simulink model "parallel_force_control_position"  (R2023a)
settings: Solver=VariableStepAuto  StartTime=0.0  StopTime=10.0  RelTol=1e-3
undefined symbols (not defined in the file): dqi, fd, K, KD, KF, KI, KP, Md, qi, robot, xd, xr
settings Model: Creator=franc  LastModifiedBy=franc

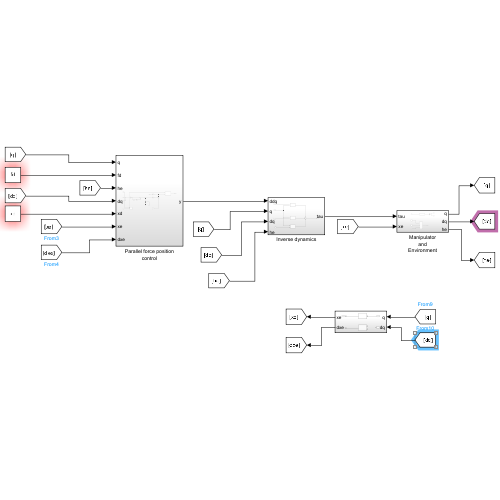
[thumbnail: Simulink's stored preview of the top-level diagram]
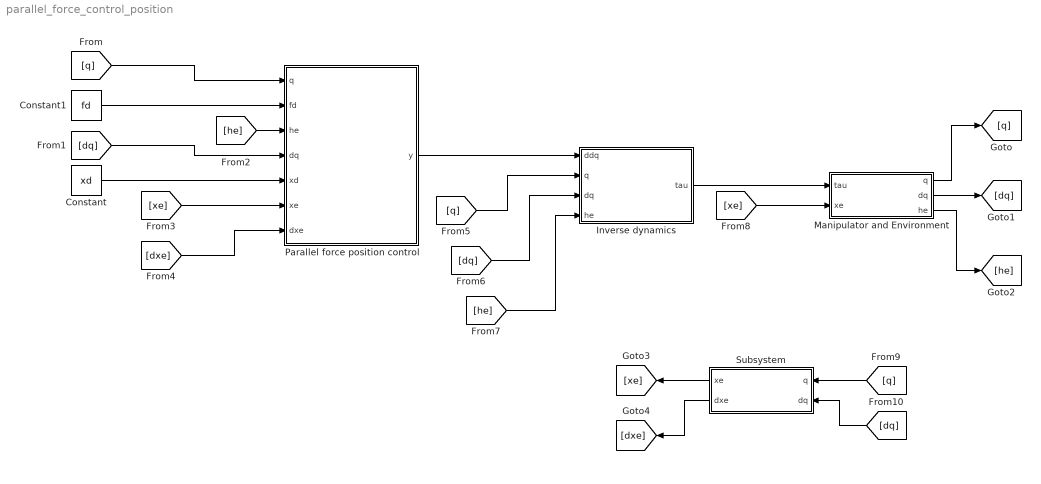
== system parallel_force_control_position ==
  Constant : Constant  Value=xd
  Constant1 : Constant  Value=fd
  Inverse dynamics : Subsystem
  Manipulator and Environment : Subsystem
  Parallel force position control : Subsystem
  Subsystem : Subsystem
  wires:
  Constant/1 -> Parallel force position control/5(xd)
  Constant1/1 -> Parallel force position control/2(fd)
  [q] -> Parallel force position control/1(q)
  [dq] -> Parallel force position control/4(dq)
  [he] -> Parallel force position control/3(he)
  [xe] -> Parallel force position control/6(xe)
  [dxe] -> Parallel force position control/7(dxe)
  Parallel force position control/1(y) -> Inverse dynamics/1(ddq)
  [q] -> Inverse dynamics/2(q)
  [dq] -> Inverse dynamics/3(dq)
  [he] -> Inverse dynamics/4(he)
  Inverse dynamics/1(tau) -> Manipulator and Environment/1(tau)
  [xe] -> Manipulator and Environment/2(xe)
  Manipulator and Environment/1(q) -> [q]
  Manipulator and Environment/2(dq) -> [dq]
  Manipulator and Environment/3(he) -> [he]
  Subsystem/1(xe) -> [xe]
  Subsystem/2(dxe) -> [dxe]
  [dq] -> Subsystem/2(dq)
  [q] -> Subsystem/1(q)

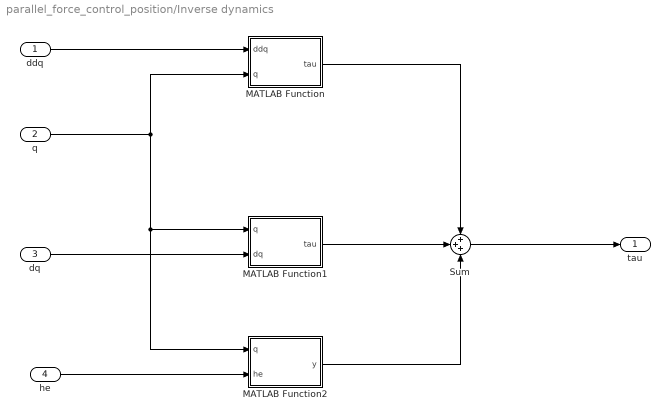
== system parallel_force_control_position/Inverse dynamics ==
  ddq : Inport
  q : Inport  Port=2
  dq : Inport  Port=3
  he : Inport  Port=4
  MATLAB Function : MATLAB Function  TreatAsAtomicUnit=on
  MATLAB Function1 : MATLAB Function  TreatAsAtomicUnit=on
  MATLAB Function2 : MATLAB Function  TreatAsAtomicUnit=on
  Sum : Sum  Inputs=+++
  tau : Outport
  wires:
  ddq/1 -> MATLAB Function/1(ddq)
  q/1 -> MATLAB Function1/1(q), MATLAB Function2/1(q), MATLAB Function/2(q)
  dq/1 -> MATLAB Function1/2(dq)
  he/1 -> MATLAB Function2/2(he)
  MATLAB Function1/1(tau) -> Sum/2
  MATLAB Function/1(tau) -> Sum/1
  MATLAB Function2/1(y) -> Sum/3
  Sum/1 -> tau/1

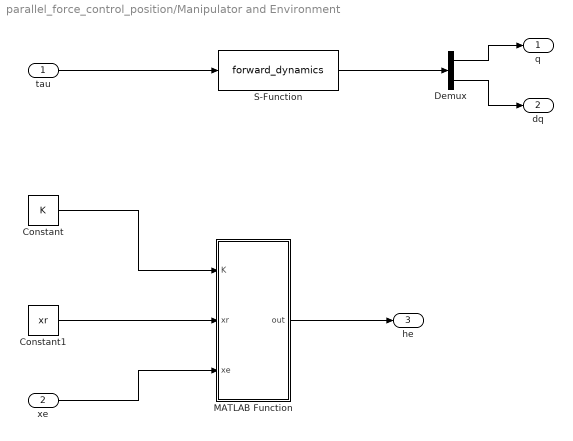
== system parallel_force_control_position/Manipulator and Environment ==
  tau : Inport
  xe : Inport  Port=2
  Constant : Constant  Value=K
  Constant1 : Constant  Value=xr
  Demux : Demux  Outputs=2
  MATLAB Function : MATLAB Function  TreatAsAtomicUnit=on
  S-Function : S-Function  FunctionName=forward_dynamics  Parameters=robot,qi,dqi  SFunctionDeploymentMode=off  EnableBusSupport=off
  q : Outport
  dq : Outport  Port=2
  he : Outport  Port=3
  wires:
  tau/1 -> S-Function/1
  Constant1/1 -> MATLAB Function/2(xr)
  Constant/1 -> MATLAB Function/1(K)
  xe/1 -> MATLAB Function/3(xe)
  MATLAB Function/1(out) -> he/1
  S-Function/1 -> Demux/1
  Demux/1 -> q/1
  Demux/2 -> dq/1

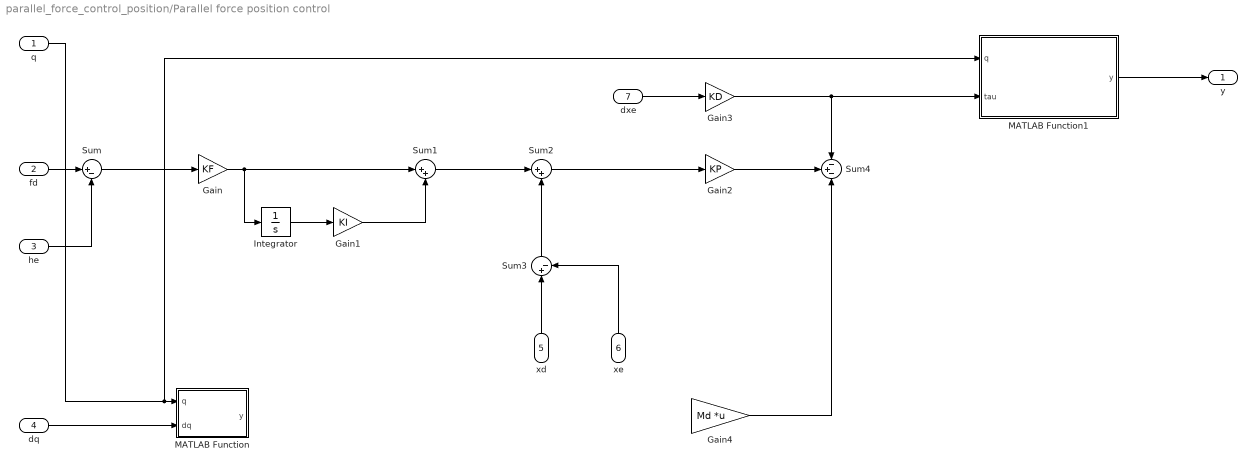
== system parallel_force_control_position/Parallel force position control ==
  q : Inport
  fd : Inport  Port=2
  he : Inport  Port=3
  dq : Inport  Port=4
  xd : Inport  Port=5
  xe : Inport  Port=6
  dxe : Inport  Port=7
  Gain : Gain  Gain=KF
  Gain1 : Gain  Gain=KI
  Gain2 : Gain  Gain=KP
  Gain3 : Gain  Gain=KD
  Gain4 : Gain  Gain=Md  Multiplication=Matrix(K*u)
  Integrator : Integrator
  MATLAB Function : MATLAB Function  TreatAsAtomicUnit=on
  MATLAB Function1 : MATLAB Function  TreatAsAtomicUnit=on
  Sum : Sum  Inputs=|+-
  Sum1 : Sum  Inputs=|++
  Sum2 : Sum  Inputs=|++
  Sum3 : Sum  Inputs=|+-
  Sum4 : Sum  Inputs=-+-
  y : Outport
  wires:
  Integrator/1 -> Gain1/1
  Gain/1 -> Sum1/1, Integrator/1
  fd/1 -> Sum/1
  Sum/1 -> Gain/1
  he/1 -> Sum/2
  Gain1/1 -> Sum1/2
  Sum1/1 -> Sum2/1
  xd/1 -> Sum3/1
  xe/1 -> Sum3/2
  Sum3/1 -> Sum2/2
  Sum2/1 -> Gain2/1
  dxe/1 -> Gain3/1
  Gain2/1 -> Sum4/2
  Gain3/1 -> MATLAB Function1/2(tau), Sum4/1
  Gain4/1 -> Sum4/3
  dq/1 -> MATLAB Function/2(dq)
  q/1 -> MATLAB Function1/1(q), MATLAB Function/1(q)
  MATLAB Function1/1(y) -> y/1

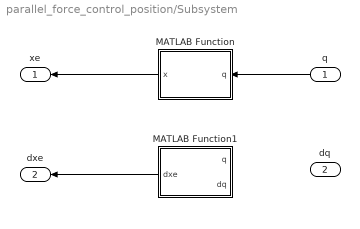
== system parallel_force_control_position/Subsystem ==
  q : Inport
  dq : Inport  Port=2
  MATLAB Function : MATLAB Function  TreatAsAtomicUnit=on
  MATLAB Function1 : MATLAB Function  TreatAsAtomicUnit=on
  xe : Outport
  dxe : Outport  Port=2
  wires:
  q/1 -> MATLAB Function/1(q)
  MATLAB Function/1(x) -> xe/1
  MATLAB Function1/1(dxe) -> dxe/1

== matlab function parallel_force_control_position/Parallel force position control/MATLAB Function ==
  data: q input; y output; dq input
function y = Ja_diff(q,dq)

y = get_derivative_Ja_as_9(q(1),q(2),q(3),dq(1),dq(2),dq(3));

== matlab function parallel_force_control_position/Inverse dynamics/MATLAB Function ==
  data: ddq input; tau output; q input
function tau = B(ddq,q)

tau = get_B_as_7(q(1),q(3))*ddq;

== matlab function parallel_force_control_position/Inverse dynamics/MATLAB Function1 ==
  data: q input; tau output; dq input
function tau = n(q,dq)


tau = get_n_as_7(q(1),q(3),dq(1),dq(3));

== matlab function parallel_force_control_position/Inverse dynamics/MATLAB Function2 ==
  data: q input; y output; he input
function y = fcn(q,he)
y = get_Ja_as_9(q(1),q(2),q(3))'*he;

== matlab function parallel_force_control_position/Manipulator and Environment/MATLAB Function ==
  data: K input; out output; xr input; xe input
function out = hde(K,xr,xe)

if xe(3)<xr(3)
    out = K*(xe-xr);
else
    out = zeros(6,1);

end

== matlab function parallel_force_control_position/Subsystem/MATLAB Function ==
  data: q input; x output
function x = fcn(q)
x = get_k_as_9(q(1),q(2),q(3));

== matlab function parallel_force_control_position/Subsystem/MATLAB Function1 ==
  data: q input; dxe output; dq input
function dxe = Ja(q,dq)

dxe = get_Ja_as_9(q(1),q(2),q(3))*dq;

== matlab function parallel_force_control_position/Parallel force position control/MATLAB Function1 ==
  data: q input; y output; tau input
function y = Ja_inverse(q,tau)


y = get_Ja_inverse_as_9(q(1),q(2),q(3))*tau;
